simulink model "disturbance_generator"  (R2015a)
settings: Solver=ode3  StartTime=0.0  StopTime=simu.time  FixedStep=0.001  RelTol=1e-3
undefined symbols (not defined in the file or in its folder): simu
settings Model: Creator=Xiaotian  LastModifiedBy=Xiaotian

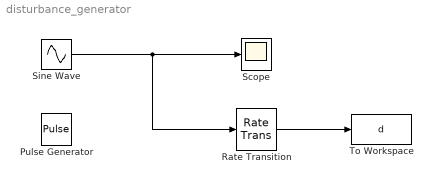
== system disturbance_generator ==
  Pulse Generator : DiscretePulseGenerator  PulseType=Time based  Amplitude=10  Period=20  PulseWidth=5
  Rate Transition : RateTransition
  Scope : Scope
      settings: YMin=-0  YMax=2
  Sine Wave : Sin  Amplitude=0.1  SampleTime=0
  To Workspace : ToWorkspace  VariableName=d  SaveFormat=Timeseries  SampleTime=simu.samlping_time
  wires:
  Rate Transition/1 -> To Workspace/1
  Sine Wave/1 -> Rate Transition/1, Scope/1
